simulink model "model"  (R2023b)
settings: Solver=VariableStepAuto  StartTime=0.0  StopTime=10  RelTol=1e-3
settings Model: Creator=student  LastModifiedBy=Jakub

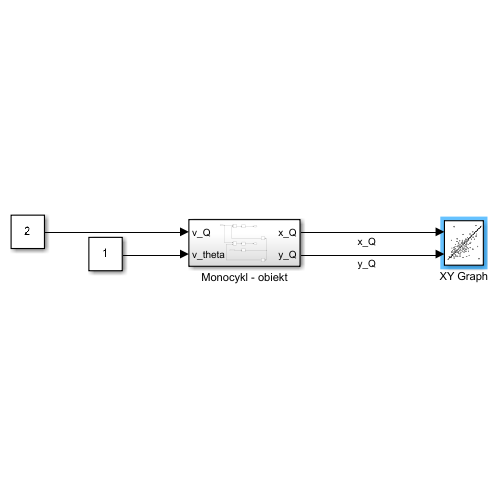
[thumbnail: Simulink's stored preview of the top-level diagram]
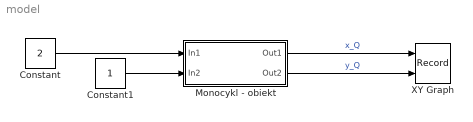
== system model ==
  Constant : Constant  Value=2
  Constant1 : Constant
  Monocykl - obiekt : Subsystem
  XY Graph : Record  FileSettingsInternal="{\"entries\":[{\"content\":{\"excelSettings\":{\"content\":{},\"type\":\"Streamout.ExcelSettings\"}},\"type\":\"Streamout.FileSettingStorage\",\"uuid\":\"\"}],\"packageUris\":[\"http:\\/\\/schema.mathworks.com\\/mf0\\/streamout_blocks\\/R2020a\"],\"version\":\"1.0\"}"  Layout=[1 1]  SignalsInternal="{\"entries\":[{\"content\":{\"signals\":[{\"content\":{\"blockPath\":[],\"dimensions\":[1],\"domain\":\"\",\"lineColor\":\"#a2142f\",\"plots\":[1],\"port\":1,\"sid\":[\"\"],\"signalID\":110,\"signalName\":\"x_Q\"},\"type\":\"RecordBlkView.Signal\",\"uuid\":\"\"},{\"content\":{\"blockPath\":[],\"dimensions\":[1],\"domain\":\"\",\"lineColor\":\"#139fff\",\"plots\":[1],\"port\":2,\"sid\":[\"\"],\"signalID\":114,\"signalName\":\"y_Q\"},\"type\":\"RecordBlkView.Signal\",\"uuid\":\"\"}]},\"type\":\"RecordBlkView.InputSignals\",\"uuid\":\"\"}],\"packageUris\":[\"http:\\/\\/schema.mathworks.com\\/mf0\\/streamout_blocks\\/R2020a\"],\"version\":\"1.0\"}"  VisualizationBindings="{\"xyplotplugin\":{\"info\":[{\"series\":[{\"bindingParametersList\":[{\"parameter\":\"X-Axis\",\"signalID\":110,\"signalName\":\"x_Q\"},{\"parameter\":\"Y-Axis\",\"signalID\":114,\"signalName\":\"y_Q\"}],\"seriesID\":9931}],\"subplotID\":1}]}}"  CompatibilityTag=XY  st=-1
  wires:
  Constant/1 -> Monocykl - obiekt/1(In1)
  Constant1/1 -> Monocykl - obiekt/2(In2)
  Monocykl - obiekt/1(Out1) -> XY Graph/1  "x_Q"
  Monocykl - obiekt/2(Out2) -> XY Graph/2  "y_Q"

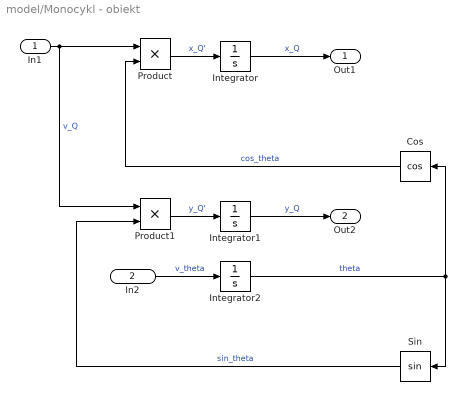
== system model/Monocykl - obiekt ==
  In1 : Inport
  In2 : Inport  Port=2
  Cos : Trigonometry  Operator=cos
  Integrator : Integrator
  Integrator1 : Integrator
  Integrator2 : Integrator
  Product : Product
  Product1 : Product
  Sin : Trigonometry
  Out1 : Outport
  Out2 : Outport  Port=2
  wires:
  Integrator2/1 -> Sin/1, Cos/1  "theta"
  Product/1 -> Integrator/1  "x_Q'"
  Product1/1 -> Integrator1/1  "y_Q'"
  In1/1 -> Product/1, Product1/1  "v_Q"
  Cos/1 -> Product/2  "cos_theta"
  Integrator/1 -> Out1/1  "x_Q"
  Sin/1 -> Product1/2  "sin_theta"
  In2/1 -> Integrator2/1  "v_theta"
  Integrator1/1 -> Out2/1  "y_Q"
